simulink model "ee463_projesi"  (R2025a)
settings: Solver=VariableStepAuto  StartTime=0.0  StopTime=5  RelTol=1e-3
libraries: spsVoltageMeasurementLib x3, spsDCMachineLib x1, spsDCVoltageSourceLib x1, spsDiodeLib x1, spsGroundLib x1, spsMosfetLib x1, spsPWMGeneratorDCDCLib x1, simulink x1, spsSeriesRLCBranchLib x1, spsThreePhaseProgrammableVoltageSourceLib x1, spsUniversalBridgeLib x1, spsCurrentMeasurementLib x1
settings Model: Creator=arday  LastModifiedBy=arday

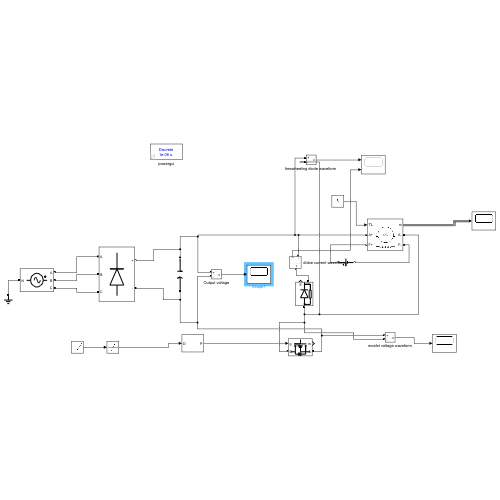
[thumbnail: Simulink's stored preview of the top-level diagram]
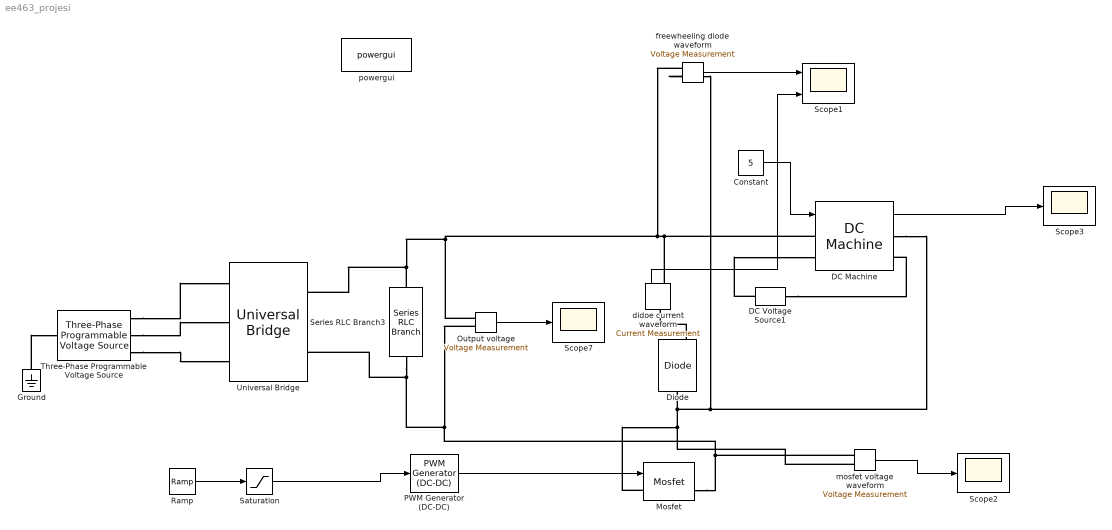
== system ee463_projesi ==
  Constant : Constant  Value=5
  DC Machine : spsDCMachineLib/DC Machine  PresetModel=No  MechanicalLoad=Torque TL  FieldType=Wound  ShowDetailedParameters=on  MeasurementBus=off  RLa=[ 1.07 0.0245]  RLf="[ 210  23]"  Laf=1.2  MachineConstant=Torque constant (N.m/A)  Ke=1.8  Kt=1.8  J=0.05  Bm=0  Tf=0  w0=1  Ifinit=1.04761904761905  TsPowergui=0  TsBlock=-1
  DC Voltage Source1 : spsDCVoltageSourceLib/DC Voltage Source  Amplitude=220  Measurements=None
  Diode : spsDiodeLib/Diode  Ron=0.02  Lon=0  Vf=1.3  IC=0  UseSnubber=0  Rs=1e5  Cs=inf  Measurements=on
  Ground : spsGroundLib/Ground  LConnTagsString=a
  Mosfet : spsMosfetLib/Mosfet  Ron=0.095  Lon=0  Rd=0.01  Vfd=1.2  IC=0  Rs=1e5  Cs=inf  Measurements=on
  Output voltage : spsVoltageMeasurementLib/Voltage Measurement  PhasorSimulation=off  OutputType=Complex  PSBequivalent=0
  PWM Generator (DC-DC) : spsPWMGeneratorDCDCLib/PWM Generator (DC-DC)  Fsw=20e3  Ts=0
  Ramp : simulink/Sources/Ramp  slope=0.2  start=0  InitialOutput=0
  Saturation : Saturate  UpperLimit=0.6  LowerLimit=-0.6
  Scope1 : Scope  NumInputPorts=2
      settings: ActiveDisplayYMinimum=-15.371601238563642  ActiveDisplayYMaximum=310.24525614035065
  Scope2 : Scope
      settings: ActiveDisplayYMinimum=-311.14396526601718  ActiveDisplayYMaximum=1.5237973821678077  DataLoggingVariableName=ScopeData2
  Scope3 : Scope
      settings: ActiveDisplayYMinimum=3.5726012997429191  ActiveDisplayYMaximum=4.5003286552658652
  Scope7 : Scope
      settings: ActiveDisplayYMinimum=293.35878266466477  ActiveDisplayYMaximum=313.53621739882431  DataLoggingVariableName=ScopeData6
  Series RLC Branch3 : spsSeriesRLCBranchLib/Series RLC Branch  LConnTagsString=__new0  RConnTagsString=__new0  BranchType=C  Resistance=1.8e-3  Inductance=1e-3  SetiL0=off  InitialCurrent=0  Capacitance=470e-6  Setx0=off  InitialVoltage=0  Measurements=None
  Three-Phase Programmable Voltage Source : spsThreePhaseProgrammableVoltageSourceLib/Three-Phase Programmable Voltage Source  PositiveSequence="[220  0 50]"  VariationEntity=None  VariationType=Table of time-amplitude pairs  VariationTypeAlt=Step  VariationStep=0.5  VariationRate=10  VariationMagnitude=0.3  VariationFrequency=2  VariationTiming=[1 2]  VariationPhaseA=off  Amplitudes=[1 0.8 1.2 1.0]  TimeValues=[0 0.1 0.15 0.2]  HarmonicGeneration=off  HarmonicA=[3 0.2 -25 0]  HarmonicB=[2 0.15 35 2]  Timing="[0.05  3]"  BusType=swing  Pref=0  Qref=0  Qmin=-inf  Qmax=inf
  Universal Bridge : spsUniversalBridgeLib/Universal Bridge  Arms=3  SnubberResistance=1e5  SnubberCapacitance=inf  Device=Diodes  Ron=0.01  Lon=0  ForwardVoltages="[  0  0  ]"  ForwardVoltage=1.1  GTOparameters=[ 10e-6 , 20e-6 ]  IGBTparameters=[ 1e-6 , 2e-6 ]  Measurements=None  Measurements_2=None  converterType=Rectifier
  "didoe current waveform " : spsCurrentMeasurementLib/Current Measurement  PhasorSimulation=off  OutputType=Complex  PSBequivalent=0
  "freewheeling diode waveform " : spsVoltageMeasurementLib/Voltage Measurement  PhasorSimulation=off  OutputType=Complex  PSBequivalent=0
  mosfet voltage waveform : spsVoltageMeasurementLib/Voltage Measurement  PhasorSimulation=off  OutputType=Complex  PSBequivalent=0
  powergui : sps_lib/powergui  Priority=1  SimulationMode=Discrete  SampleTime=1e-6  frequency=60  Iterations=50  frequencyindice=0  Pbase=100e6  ErrMax=1e-4  UnitsV=kV  UnitsW=MW  buscounter=0  FunctionMessages=off  echomessages=off  EnableUseOfTLC=off  CurrentSourceSwitches=off  DisableSnubberDevices=off  DisableRonSwitches=off  DisableVfSwitches=off  DisplayEquations=off  AutomaticDiscreteSolvers=off  SolverType=Tustin/Backward Euler (TBE)  Interpol=off  ExternalGateDelay=off  methode=off  Ts=100  x0status=blocks  SPID=on  SwTol=0  HookPort=off  NonlinearTolerance=1e-4  nMaxIteration=100  ContinueOnMaxIteration=off  RestoreLinks=warning  ResistiveCurrentMeasurement=off  Frange=[0:2:500]  Ylog=off  Xlog=on  ShowGrid=off  save=off  variable=ZData  structure=0  ZoomFFT=off  StartTime=0.0  cycles=1  DisplayStyle=1  fundamental=60  FreqAxis=off  MaxFrequency=1000  frequencyindicesteady=1  RmsSteady=1  display=off
  wires:
  Output voltage/1 -> Scope7/1
  PWM Generator (DC-DC)/1 -> Mosfet/1
  Constant/1 -> DC Machine/1
  DC Machine/1 -> Scope3/1
  Ramp/1 -> Saturation/1
  Saturation/1 -> PWM Generator (DC-DC)/1
  "freewheeling diode waveform "/1 -> Scope1/1
  mosfet voltage waveform/1 -> Scope2/1
  "didoe current waveform "/1 -> Scope1/2
  connections:
  Series RLC Branch3/RConn1 -- Mosfet/RConn1 -- mosfet voltage waveform/LConn1 -- Output voltage/LConn2 -- Universal Bridge/RConn2
  Series RLC Branch3/LConn1 -- DC Machine/LConn1 -- "didoe current waveform "/RConn1 -- "freewheeling diode waveform "/LConn1 -- Output voltage/LConn1 -- Universal Bridge/RConn1
  DC Voltage Source1/RConn1 -- DC Machine/LConn2
  DC Voltage Source1/LConn1 -- DC Machine/RConn2
  Three-Phase Programmable Voltage Source/RConn1 -- Universal Bridge/LConn1
  Three-Phase Programmable Voltage Source/RConn2 -- Universal Bridge/LConn2
  Three-Phase Programmable Voltage Source/RConn3 -- Universal Bridge/LConn3
  Ground/LConn1 -- Three-Phase Programmable Voltage Source/LConn1
  DC Machine/RConn1 -- Mosfet/LConn1 -- mosfet voltage waveform/LConn2 -- Diode/LConn1 -- "freewheeling diode waveform "/LConn2
  Diode/RConn1 -- "didoe current waveform "/LConn1
